simulink model "Wood_Berry_mf_desacopladorEE"  (R2020b)
settings: Solver=VariableStepAuto  StartTime=0.0  StopTime=100  MaxStep=1e-3  MinStep=1e-4  RelTol=1e-3
values from neighbouring files (symbols this model uses):
  Kc11_DE = Gm/2.2    [Wood_Berry.m]
  Kc22_McAv = Kc22*(Lambda(2,2) - sqrt(Lambda(2,2)^2 - Lambda(2,2)))    [Wood_Berry.m]
  ti11_DE = (2*pi()/Wcg)/1.2    [Wood_Berry.m]
undefined symbols (not defined in the file or in its folder): ti22
libraries: cstblocks x8, pid_lib x2
settings Model: Creator=Gustavo Caldas  LastModifiedBy=Gustavo Caldas

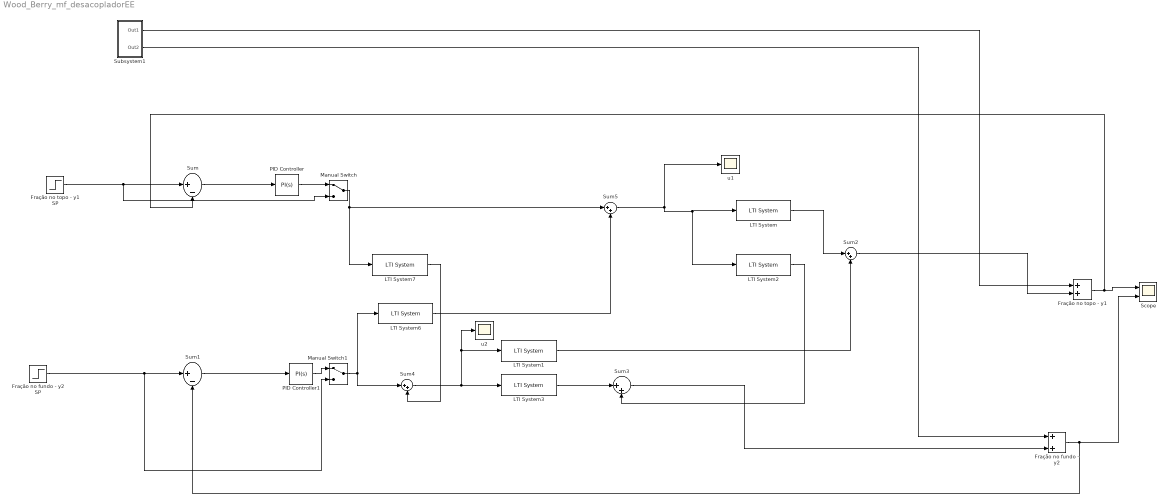
== system Wood_Berry_mf_desacopladorEE ==
  Fração no fundo - y2 : Sum
  Fração no fundo - y2 SP : Step  Time=0  SampleTime=0
  Fração no topo - y1 : Sum
  Fração no topo - y1 SP : Step  Time=0  After=0  SampleTime=0
  LTI System : cstblocks/LTI System  sys=tf11  IC=[]
  LTI System1 : cstblocks/LTI System  sys=tf12  IC=[]
  LTI System2 : cstblocks/LTI System  sys=tf21  IC=[]
  LTI System3 : cstblocks/LTI System  sys=tf22  IC=[]
  LTI System6 : cstblocks/LTI System  sys=Gl1_EE  IC=[]
  LTI System7 : cstblocks/LTI System  sys=Gl2_EE  IC=[]
  Manual Switch : ManualSwitch
  Manual Switch1 : ManualSwitch
  PID Controller : pid_lib/PID Controller  Controller=PI  Form=Ideal  TimeDomain=Continuous-time  UseExternalTs=off  SampleTime=-1  IntegratorMethod=Forward Euler  FilterMethod=Forward Euler  ControllerParametersSource=internal  P=Kc11_DE  I=1/ti11_DE  D=1  UseFilter=on  N=100  TunerSelectOption=Transfer Function Based (PID Tuner App)  InitialConditionSource=internal  InitialConditionForIntegrator=0  InitialConditionForFilter=0  DifferentiatorICPrevScaledInput=0  ExternalReset=none  TrackingMode=off  Kt=1  LimitOutput=off  SatLimitsSource=internal  UpperSaturationLimit=inf  LowerSaturationLimit=-inf  LinearizeAsGain=on  AntiWindupMode=none  Kb=1  POutMin=[]  POutMax=[]  IOutMin=[]  IOutMax=[]  DOutMin=[]  DOutMax=[]  NOutMin=[]  NOutMax=[]  SumOutMin=[]  SumOutMax=[]  SaturationOutMin=[]  SaturationOutMax=[]  PParamMin=[]  PParamMax=[]  IParamMin=[]  IParamMax=[]  DParamMin=[]  DParamMax=[]  NParamMin=[]  NParamMax=[]  KbParamMin=[]  KbParamMax=[]  KtParamMin=[]  KtParamMax=[]  KbOutMin=[]  KbOutMax=[]  KtOutMin=[]  KtOutMax=[]  IntegratorOutMin=[]  IntegratorOutMax=[]  FilterOutMin=[]  FilterOutMax=[]  SumI1OutMin=[]  SumI1OutMax=[]  SumI2OutMin=[]  SumI2OutMax=[]  SumI3OutMin=[]  SumI3OutMax=[]  SumI4OutMin=[]  SumI4OutMax=[]  SumDOutMin=[]  SumDOutMax=[]  DifferentiatorOutMin=[]  DifferentiatorOutMax=[]  FilterDiffOutCoefMin=[]  FilterDiffOutCoefMax=[]  ReciprocalOutMin=[]  ReciprocalOutMax=[]  SumDenOutMin=[]  SumDenOutMax=[]  SumNumOutMin=[]  SumNumOutMax=[]  DivideOutMin=[]  DivideOutMax=[]  UdiffTsProdOutMin=[]  UdiffTsProdOutMax=[]  NTsProdOutMin=[]  NTsProdOutMax=[]  UintegralTsProdOutMin=[]  UintegralTsProdOutMax=[]  UngainTsProdOutMin=[]  UngainTsProdOutMax=[]  IntegratorContinuousStateAttributes=''  IntegratorStateMustResolveToSignalObject=off  IntegratorRTWStateStorageClass=Auto  FilterContinuousStateAttributes=''  FilterStateMustResolveToSignalObject=off  FilterRTWStateStorageClass=Auto  ParallelPVariant=Passthrough  IdealPVariant=InternalParameters  IVariant=InternalParameters  DVariant=Disabled  IntegratorVariant=Continuous  SatVariant=Disabled  AWVariant=Passthrough  PCopyVariant=Disabled  TRVariant=Disabled  FdbkBlocksVariant=Forward  IdealPFdbkVariant=Disabled  SatFdbkVariant=Disabled  DerivativeFilterVariant=Disabled  NVariant=Disabled  NCopyVariant=Disabled_SignalSpec  FilterICVariant=Disabled  IntegratorICVariant=InternalICs  ExternalResetVariant=Disabled  TRSumVariant=Passthrough  SumFdbkVariant=Disabled  SumVariant=Sum_PI  TsampFilterVariant=InternalTs  TsampNgainVariant=Passthrough  TsampIntegralVariant=Passthrough  ExternalSaturationOutDataTypeStr=Inherit: Same as second input
  PID Controller1 : pid_lib/PID Controller  Controller=PI  Form=Ideal  TimeDomain=Continuous-time  UseExternalTs=off  SampleTime=-1  IntegratorMethod=Forward Euler  FilterMethod=Forward Euler  ControllerParametersSource=internal  P=Kc22_McAv  I=1/ti22  D=0  UseFilter=on  N=100  TunerSelectOption=Transfer Function Based (PID Tuner App)  InitialConditionSource=internal  InitialConditionForIntegrator=0  InitialConditionForFilter=0  DifferentiatorICPrevScaledInput=0  ExternalReset=none  TrackingMode=off  Kt=1  LimitOutput=off  SatLimitsSource=internal  UpperSaturationLimit=inf  LowerSaturationLimit=-inf  LinearizeAsGain=on  AntiWindupMode=none  Kb=1  POutMin=[]  POutMax=[]  IOutMin=[]  IOutMax=[]  DOutMin=[]  DOutMax=[]  NOutMin=[]  NOutMax=[]  SumOutMin=[]  SumOutMax=[]  SaturationOutMin=[]  SaturationOutMax=[]  PParamMin=[]  PParamMax=[]  IParamMin=[]  IParamMax=[]  DParamMin=[]  DParamMax=[]  NParamMin=[]  NParamMax=[]  KbParamMin=[]  KbParamMax=[]  KtParamMin=[]  KtParamMax=[]  KbOutMin=[]  KbOutMax=[]  KtOutMin=[]  KtOutMax=[]  IntegratorOutMin=[]  IntegratorOutMax=[]  FilterOutMin=[]  FilterOutMax=[]  SumI1OutMin=[]  SumI1OutMax=[]  SumI2OutMin=[]  SumI2OutMax=[]  SumI3OutMin=[]  SumI3OutMax=[]  SumI4OutMin=[]  SumI4OutMax=[]  SumDOutMin=[]  SumDOutMax=[]  DifferentiatorOutMin=[]  DifferentiatorOutMax=[]  FilterDiffOutCoefMin=[]  FilterDiffOutCoefMax=[]  ReciprocalOutMin=[]  ReciprocalOutMax=[]  SumDenOutMin=[]  SumDenOutMax=[]  SumNumOutMin=[]  SumNumOutMax=[]  DivideOutMin=[]  DivideOutMax=[]  UdiffTsProdOutMin=[]  UdiffTsProdOutMax=[]  NTsProdOutMin=[]  NTsProdOutMax=[]  UintegralTsProdOutMin=[]  UintegralTsProdOutMax=[]  UngainTsProdOutMin=[]  UngainTsProdOutMax=[]  IntegratorContinuousStateAttributes=''  IntegratorStateMustResolveToSignalObject=off  IntegratorRTWStateStorageClass=Auto  FilterContinuousStateAttributes=''  FilterStateMustResolveToSignalObject=off  FilterRTWStateStorageClass=Auto  ParallelPVariant=Passthrough  IdealPVariant=InternalParameters  IVariant=InternalParameters  DVariant=Disabled  IntegratorVariant=Continuous  SatVariant=Disabled  AWVariant=Passthrough  PCopyVariant=Disabled  TRVariant=Disabled  FdbkBlocksVariant=Forward  IdealPFdbkVariant=Disabled  SatFdbkVariant=Disabled  DerivativeFilterVariant=Disabled  NVariant=Disabled  NCopyVariant=Disabled_SignalSpec  FilterICVariant=Disabled  IntegratorICVariant=InternalICs  ExternalResetVariant=Disabled  TRSumVariant=Passthrough  SumFdbkVariant=Disabled  SumVariant=Sum_PI  TsampFilterVariant=InternalTs  TsampNgainVariant=Passthrough  TsampIntegralVariant=Passthrough  ExternalSaturationOutDataTypeStr=Inherit: Same as second input
  Scope : Scope  NumInputPorts=2
  Subsystem1 : Subsystem
  Sum : Sum  Inputs=|+-
  Sum1 : Sum  Inputs=|+-
  Sum{2..5} (4 alike) : Sum  Inputs=|++
  u1 : Scope
  u2 : Scope
  wires:
  Fração no topo - y1/1 -> Scope/1, Sum/2
  Fração no fundo - y2/1 -> Scope/2, Sum1/2
  Subsystem1/2(Out2) -> Fração no fundo - y2/1
  Subsystem1/1(Out1) -> Fração no topo - y1/1
  LTI System1/1 -> Sum2/2
  Sum4/1 -> LTI System1/1, u2/1, LTI System3/1
  Manual Switch1/1 -> LTI System6/1, Sum4/1
  Sum3/1 -> Fração no fundo - y2/2
  LTI System/1 -> Sum2/1
  LTI System7/1 -> Sum4/2
  Sum1/1 -> PID Controller1/1
  Fração no fundo - y2 SP/1 -> Manual Switch1/2, Sum1/1
  PID Controller1/1 -> Manual Switch1/1
  LTI System3/1 -> Sum3/1
  LTI System2/1 -> Sum3/2
  LTI System6/1 -> Sum5/2
  Sum2/1 -> Fração no topo - y1/2
  Sum/1 -> PID Controller/1
  Sum5/1 -> u1/1, LTI System/1, LTI System2/1
  PID Controller/1 -> Manual Switch/1
  Manual Switch/1 -> LTI System7/1, Sum5/1
  Fração no topo - y1 SP/1 -> Sum/1, Manual Switch/2

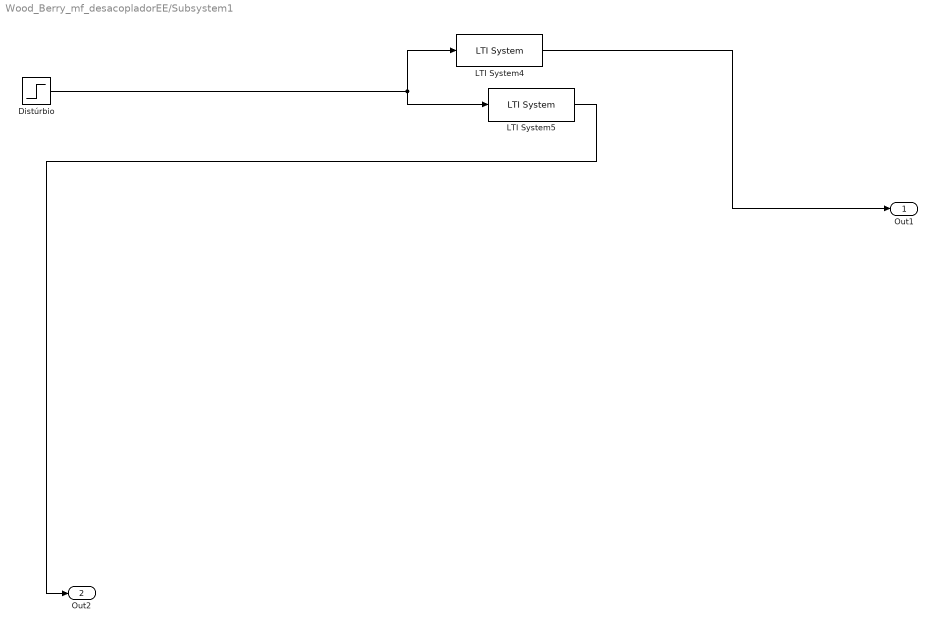
== system Wood_Berry_mf_desacopladorEE/Subsystem1 ==
  Distúrbio : Step  Time=0  After=0  SampleTime=0
  LTI System4 : cstblocks/LTI System  sys=tfd1  IC=[]
  LTI System5 : cstblocks/LTI System  sys=tfd2  IC=[]
  Out1 : Outport
  Out2 : Outport  Port=2
  wires:
  Distúrbio/1 -> LTI System5/1, LTI System4/1
  LTI System4/1 -> Out1/1
  LTI System5/1 -> Out2/1
